simulink model "model2"  (R2024a)
settings: Solver=VariableStepAuto  StartTime=0.0  StopTime=10.0  RelTol=1e-5
values from neighbouring files (symbols this model uses):
  a0 = -2    [script2.m]
  a1 = 1    [script2.m]
  a2 = 1    [script2.m]
  k0 = -15    [script2.m]
  k1 = -1.5    [script2.m]
  T = 0.5    [script2.m]
settings Model: Creator=eva  LastModifiedBy=eva

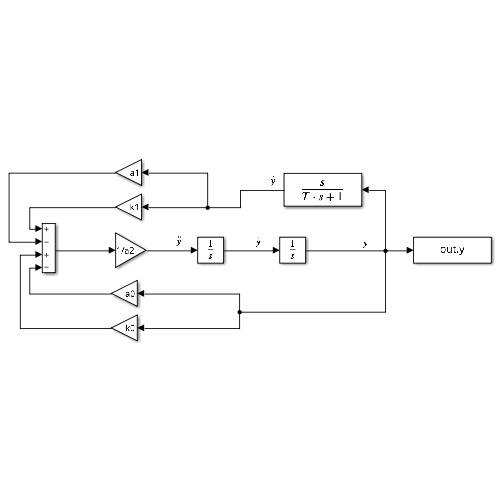
[thumbnail: Simulink's stored preview of the top-level diagram]
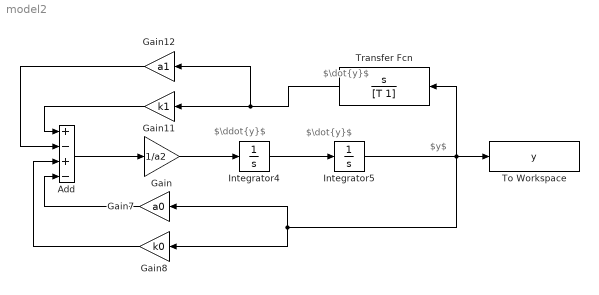
== system model2 ==
  note: $\dot{y}$
  note: $y$
  note: $\ddot{y}$
  note: $\dot{y}$
  Add : Sum  Inputs=+-+-
  Gain : Gain  Gain=1/a2
  Gain11 : Gain  Gain=k1
  Gain12 : Gain  Gain=a1
  Gain7 : Gain  Gain=a0
  Gain8 : Gain  Gain=k0
  Integrator4 : Integrator  InitialCondition=-1
  Integrator5 : Integrator
  To Workspace : ToWorkspace  VariableName=y  SaveFormat=Structure With Time  SampleTime=-1
  Transfer Fcn : TransferFcn  Numerator=[1 0]  Denominator=[T 1]
  wires:
  Add/1 -> Gain/1
  Integrator4/1 -> Integrator5/1
  Gain7/1 -> Add/4
  Gain12/1 -> Add/2
  Gain8/1 -> Add/3
  Gain11/1 -> Add/1
  Integrator5/1 -> Gain7/1, Gain8/1, To Workspace/1, Transfer Fcn/1
  Transfer Fcn/1 -> Gain11/1, Gain12/1
  Gain/1 -> Integrator4/1
